simulink model "Citation_FlightGear_v2"  (R2026a)
settings: Solver=ode5  StopTime=40  FixedStep=0.01  EnableMultiTasking=on
InitFcn:
  | run('initcit.m')
  | run('id_init.m')
values from neighbouring files (symbols this model uses):
  cv1 = 20000    [gear_params.m]
  cv2 = cv1    (= 20000)    [gear_params.m]
  cv3 = 4000    [gear_params.m]
  cv4 = 20000    [gear_params.m]
  deltagmax1 = 0.25    [gear_params.m]
  deltagmax2 = deltagmax1    (= 0.25)    [gear_params.m]
  deltagmax3 = 0.24    [gear_params.m]
  deltagmax4 = 0.02    [gear_params.m]
  kt1 = 525020    [gear_params.m]
  kt2 = kt1    (= 525020)    [gear_params.m]
  kt3 = 457050    [gear_params.m]
  murol = 0.03*10    (= 0.3)    [gear_params.m]
  P1 = 2000    [gear_params.m]
  P2 = P1    (= 2000)    [gear_params.m]
  P3 = 2550    [gear_params.m]
  P4 = 40000    [gear_params.m]
  PL0 = 10000*eye(6)    [id_init.m]
  PM0 = 10000*eye(4)    [id_init.m]
  PN0 = 10000*eye(6)    [id_init.m]
  PX0 = 10000*eye(5)    [id_init.m]
  PY0 = 10000*eye(6)    [id_init.m]
  PZ0 = 10000*eye(4)    [id_init.m]
  thetaL0 = zeros(6,1)    [id_init.m]
  thetaM0 = zeros(4,1)    [id_init.m]
  thetaN0 = zeros(6,1)    [id_init.m]
  thetaX0 = zeros(5,1)    [id_init.m]
  thetaY0 = zeros(6,1)    [id_init.m]
  thetaZ0 = zeros(4,1)    [id_init.m]
  TL = 7.0875e-06    [id_init.m]    (also in plot_comparison_step_4.m = T_var(4))
  TM = 3.2564e-06    [id_init.m]    (also in plot_comparison_step_4.m = T_var(5))
  TN = 5.4692e-07    [id_init.m]    (also in plot_comparison_step_4.m = T_var(6))
  TX = 2.2784e-06    [id_init.m]    (also in plot_comparison_step_4.m = T_var(1))
  TY = 8.0633e-07    [id_init.m]    (also in plot_comparison_step_4.m = T_var(2))
  TZ = 2.8004e-05    [id_init.m]    (also in plot_comparison_step_4.m = T_var(3))
  xl1 = xcg-6.858    [gear_params.m]
  xl2 = xcg-6.858    [gear_params.m]
  xl3 = xcg-2.0752    [gear_params.m]
  xl4 = xcg-12.742    [gear_params.m]
  yl1 = 1.918    [gear_params.m]
  yl2 = -1.918    [gear_params.m]
  yl3 = 0    [gear_params.m]
  yl4 = 0    [gear_params.m]
  zl1 = zcg-1.701    [gear_params.m]
  zl2 = zcg-1.701    [gear_params.m]
  zl3 = zcg-1.7488    [gear_params.m]
  zl4 = zcg-2.78    [gear_params.m]
undefined symbols (not defined in the file or in its folder): chord, Deng, ealphag, ealphas, g0, hDME, hGS, lh, massinit, matbuaf, matdaf, matdam, matdbbf, matdeaf, matdgaf, matdqaf, matduaf, matdwaw, matedhr, mateif, matelhr, matemhr, matemv1, matemv2, matemve, matetam, mateuaf, matfaaf, matfaxl, matff, matibaf, matibb, matibmh, matipaf, matipmh, matiraf, matiuaf, matiwaf, matlaf, matlam, matleaf, matleam, matlgaf, matlqaf, matluaf, matmaaf, matmaam, matmaf, matmam, matmbbf, matmeaf, matmeam, matmgaf, matmqaf, matmrbr, matn1d, matn2d, matnbab, matnbaf, matnbmh ... (+53)
libraries: simulink x12, aerolibfltsims x3, aerolibconvert2 x2, aerolibobsolete x1, aerolibanimutils x1
(part 4 of 5)

== system Citation_FlightGear_v2/Cessna Citation 500/Citation model DASMAT/AIRCRAFT MODEL/AFM/Aeromod/SubSystem/model/CLLCAL ==
  in_1 : Inport
  Abs : Abs
  CIBAB : Subsystem  mask(3-D Table Lookup){xindex=matibb(2:5,1), yindex=matibb(1,2:4), zindex=matibb(1,5:7), table=matibb(2:5,2:10)}
      mask prompts: xindex "X Index"; yindex "Y Index"; zindex "Z Index"
      mask help:
      | Three Dimensional Table Lookup
      | The first, second and third input corresponds to the X,Y and Z Index
      mask Help: This block returns a linearly interpolated intersection from the table using the X index (which corresponds to the rows of the table), the Y index (which corresponds to the columns of the table) and the Z index.  Extrapolation is used.
      mask Display: plot(-10,-10,110,110,[90,50,10],[90,40,30],[90,50,10],[50,26,20],[90,50,10],[22,13,10])
  CIBAF : Lookup2D  RowIndex=matibaf(2:4,1)  ColumnIndex=matibaf(1,2:4)  Table=matibaf(2:4,2:4)
  CIBMH : Lookup2D  RowIndex=matibmh(2:10,1)  ColumnIndex=matibmh(1,2:10)  Table=matibmh(2:10,2:10)
  CIPAF : Lookup2D  RowIndex=matipaf(2:3,1)  ColumnIndex=matipaf(1,2:3)  Table=matipaf(2:3,2:3)
  CIPMH : Lookup2D  RowIndex=matipmh(2:10,1)  ColumnIndex=matipmh(1,2:10)  Table=matipmh(2:10,2:10)
  CIRAF : Lookup2D  RowIndex=matiraf(2:4,1)  ColumnIndex=matiraf(1,2:4)  Table=matiraf(2:4,2:4)
  CIRUAF : Lookup2D  RowIndex=matiuaf(2:3,1)  ColumnIndex=matiuaf(1,2:3)  Table=matiuaf(2:3,2:3)
  CIRUMH : Lookup2D  RowIndex=matrumh(2:10,1)  ColumnIndex=matrumh(1,2:10)  Table=matrumh(2:10,2:10)
  CIWAF : Lookup2D  RowIndex=matiwaf(2:3,1)  ColumnIndex=matiwaf(1,2:3)  Table=matiwaf(2:3,2:3)
  CIWTAM : Lookup2D  RowIndex=matwtam(2:3,1)  ColumnIndex=matwtam(1,2:3)  Table=matwtam(2:3,2:3)
  CLL : Sum  Inputs=+++++++  InputSameDT=on  SaturateOnIntegerOverflow=on  OutDataTypeStr=Inherit: Same as first input
  CLLB : Product  InputSameDT=on  SaturateOnIntegerOverflow=on  OutDataTypeStr=Inherit: Same as first input
  CLLDA : Product  InputSameDT=on  SaturateOnIntegerOverflow=on  OutDataTypeStr=Inherit: Same as first input
  CLLDR : Product  InputSameDT=on  SaturateOnIntegerOverflow=on  OutDataTypeStr=Inherit: Same as first input
  CLLGE : Product  Inputs=3  InputSameDT=on  SaturateOnIntegerOverflow=on  OutDataTypeStr=Inherit: Same as first input
  CLLGUST : Mux  Inputs=8
  CLLP : Product  InputSameDT=on  SaturateOnIntegerOverflow=on  OutDataTypeStr=Inherit: Same as first input
  CLLR : Product  InputSameDT=on  SaturateOnIntegerOverflow=on  OutDataTypeStr=Inherit: Same as first input
  CLLTRIM : Product  InputSameDT=on  SaturateOnIntegerOverflow=on  OutDataTypeStr=Inherit: Same as first input
  Demux1 : Demux  Outputs=[1 1 1 1 1 1 1 1 1 1 1 1 1 1 1 1 1 1]
      settings: DisplayOption=none
  LFACT : Subsystem
  LROLL : Lookup  InputValues=mateif(1,:)  Table=mateif(2,:)
  Sum : Sum  Inputs=+++  InputSameDT=on  SaturateOnIntegerOverflow=on  OutDataTypeStr=Inherit: Same as first input
  Sum1 : Sum  InputSameDT=on  SaturateOnIntegerOverflow=on  OutDataTypeStr=Inherit: Same as first input
  Sum2 : Sum  InputSameDT=on  SaturateOnIntegerOverflow=on  OutDataTypeStr=Inherit: Same as first input
  Terminator_{1..7} (7 alike) : Terminator
  "neg " : Gain  Gain=-1  SaturateOnIntegerOverflow=on  OutDataTypeStr=Inherit: Same as input  ParamDataTypeStr=Inherit: Same as input
  zero : Constant  Value=0
  out_1 : Outport
  out_2 : Outport  Port=2
  wires:
  Demux1/18 -> Terminator_7/1
  Demux1/16 -> Terminator_6/1
  Demux1/15 -> Terminator_5/1
  Demux1/13 -> Terminator_4/1
  Demux1/11 -> Terminator_3/1
  Demux1/8 -> Terminator_2/1
  Demux1/2 -> Terminator_1/1
  Sum/1 -> CLLGUST/3, CLLB/2
  LFACT/1(LFACT) -> CLLGE/3
  LROLL/1 -> CLLGE/2
  CLL/1 -> out_1/1
  CLLB/1 -> CLL/1
  CIWTAM/1 -> CLLTRIM/2
  CIWAF/1 -> CLLDA/2
  Sum1/1 -> CLLDR/2
  CIRUMH/1 -> Sum1/2
  Abs/1 -> CIBAB/1(x0)
  CIRUAF/1 -> Sum1/1
  CIBAF/1 -> Sum/1
  CIPAF/1 -> Sum2/1
  CIPMH/1 -> Sum2/2
  Demux1/14 -> CIBAF/1, CIRUAF/1, CIRAF/1, LROLL/1, CIPAF/1, CIWAF/1, CIBAB/3(z0)
  Demux1/5 -> CLLB/1, Abs/1, CLLGE/1
  Demux1/4 -> CIWAF/2, CIRUAF/2, CIPAF/2, CIRAF/2, CIWTAM/2, CIBAB/2(y0), CIBAF/2
  zero/1 -> CLLGUST/2, CLLGUST/5, CLLGUST/6, CLLGUST/4, CLLGUST/1
  CLLGUST/1 -> out_2/1
  CIRAF/1 -> "neg "/1, CLLR/2
  Sum2/1 -> CLLGUST/8, CLLP/2
  "neg "/1 -> CLLGUST/7
  in_1/1 -> Demux1/1
  CLLGE/1 -> CLL/7
  CLLR/1 -> CLL/6
  CLLTRIM/1 -> CLL/4
  CLLDA/1 -> CLL/2
  Demux1/12 -> CLLTRIM/1
  Demux1/10 -> CLLDR/1
  Demux1/9 -> CLLDA/1
  Demux1/1 -> CLLP/1
  Demux1/3 -> CLLR/1
  CIBMH/1 -> Sum/2
  CIBAB/1(out_1) -> Sum/3
  Demux1/17 -> CIRUMH/2, CIWTAM/1, CIPMH/2, CIBMH/2
  Demux1/6 -> CIRUMH/1, CIPMH/1, CIBMH/1
  Demux1/7 -> LFACT/1(hcg)
  CLLP/1 -> CLL/5
  CLLDR/1 -> CLL/3

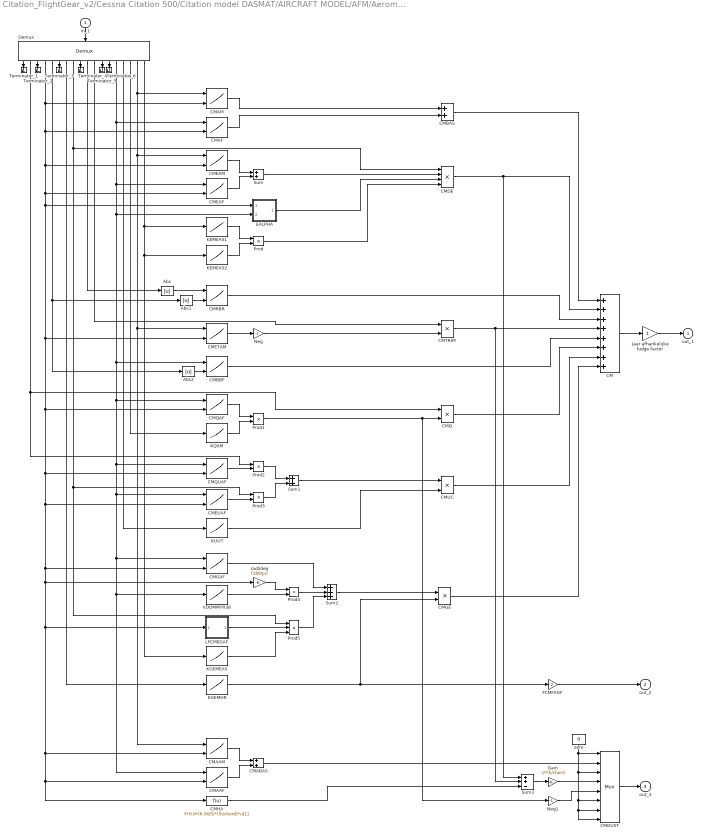
== system Citation_FlightGear_v2/Cessna Citation 500/Citation model DASMAT/AIRCRAFT MODEL/AFM/Aeromod/SubSystem/model/CMCAL ==
  in_1 : Inport
  Abs : Abs
  Abs1 : Abs
  Abs2 : Abs
  CM : Sum  Inputs=++++++++  InputSameDT=on  SaturateOnIntegerOverflow=on  OutDataTypeStr=Inherit: Same as first input
  CMAAF : Lookup2D  RowIndex=matmaaf(2:22,1)  ColumnIndex=matmaaf(1,2:22)  Table=matmaaf(2:22,2:22)
  CMAAM : Lookup2D  RowIndex=matmaam(2:22,1)  ColumnIndex=matmaam(1,2:22)  Table=matmaam(2:22,2:22)
  CMABAS : Sum  InputSameDT=on  SaturateOnIntegerOverflow=on  OutDataTypeStr=Inherit: Same as first input
  CMAF : Lookup2D  RowIndex=matmaf(2:23,1)  ColumnIndex=matmaf(1,2:23)  Table=matmaf(2:23,2:23)
  "CMAM " : Lookup2D  RowIndex=matmam(2:23,1)  ColumnIndex=matmam(1,2:23)  Table=matmam(2:23,2:23)
  CMBAS : Sum  InputSameDT=on  SaturateOnIntegerOverflow=on  OutDataTypeStr=Inherit: Same as first input
  CMBBF : Lookup2D  RowIndex=matmbbf(2:18,1)  ColumnIndex=matmbbf(1,2:18)  Table=matmbbf(2:18,2:18)
  CMDE : Product  Inputs=4  InputSameDT=on  SaturateOnIntegerOverflow=on  OutDataTypeStr=Inherit: Same as first input
  CMEAF : Lookup2D  RowIndex=matmeaf(2:23,1)  ColumnIndex=matmeaf(1,2:23)  Table=matmeaf(2:23,2:23)
  CMEAM : Lookup2D  RowIndex=matmeam(2:23,1)  ColumnIndex=matmeam(1,2:23)  Table=matmeam(2:23,2:23)
  CMETAM : Lookup2D  RowIndex=matetam(2:3,1)  ColumnIndex=matetam(1,2:3)  Table=matetam(2:3,2:3)
  CMEUAF : Lookup2D  RowIndex=mateuaf(2:23,1)  ColumnIndex=mateuaf(1,2:23)  Table=mateuaf(2:23,2:23)
  CMGAF : Lookup2D  RowIndex=matmgaf(2:4,1)  ColumnIndex=matmgaf(1,2:4)  Table=matmgaf(2:4,2:4)
  CMGE : Product  InputSameDT=on  SaturateOnIntegerOverflow=on  OutDataTypeStr=Inherit: Same as first input
  CMGUST : Mux  Inputs=8
  CMHA : Fcn  Expr=5*0.9*(6.56/S)*(lh/chord)*u[1]
  CMQ : Product  InputSameDT=on  SaturateOnIntegerOverflow=on  OutDataTypeStr=Inherit: Same as first input
  CMQAF : Lookup2D  RowIndex=matmqaf(2:23,1)  ColumnIndex=matmqaf(1,2:23)  Table=matmqaf(2:23,2:23)
  CMQUAF : Lookup2D  RowIndex=matquaf(2:23,1)  ColumnIndex=matquaf(1,2:23)  Table=matquaf(2:23,2:23)
  CMRBR : Lookup2D  RowIndex=matmrbr(2:3,1)  ColumnIndex=matmrbr(1,2:3)  Table=matmrbr(2:3,2:3)
  CMTRIM : Product  InputSameDT=on  SaturateOnIntegerOverflow=on  OutDataTypeStr=Inherit: Same as first input
  CMUC : Product  InputSameDT=on  SaturateOnIntegerOverflow=on  OutDataTypeStr=Inherit: Same as first input
  Demux : Demux  Outputs=[1 1 1 1 1 1 1 1 1 1 1 1 1 1 1 1 1 1]
      settings: DisplayOption=none
  EALPHA : Subsystem
  FCMFAGF : Gain  Gain=-2  SaturateOnIntegerOverflow=on  OutDataTypeStr=Inherit: Same as input  ParamDataTypeStr=Inherit: Same as input
  Gain : Gain  Gain=-2*lh/chord  SaturateOnIntegerOverflow=on  OutDataTypeStr=Inherit: Same as input  ParamDataTypeStr=Inherit: Same as input
  Jaar afhankelijke fudge factor : Gain
  KEMEAS1 : Lookup  InputValues=matemv1(1,:)  Table=matemv1(2,:)
  KEMEAS2 : Lookup  InputValues=matemv2(1,:)  Table=matemv2(2,:)
  KGEMEAS : Lookup  InputValues=matemve(1,:)  Table=matemve(2,:)
  KGEMHR : Lookup  InputValues=matemhr(1,:)  Table=matemhr(2,:)
  KQXM : Lookup  InputValues=matqxm(1,:)  Table=matqxm(2,:)
  KUUT : Lookup  InputValues=matuut(1,:)  Table=matuut(2,:)
  LFCMEGAF : Subsystem
  "Neg " : Gain  Gain=-1  SaturateOnIntegerOverflow=on  OutDataTypeStr=Inherit: Same as input  ParamDataTypeStr=Inherit: Same as input
  Neg1 : Gain  Gain=-1  SaturateOnIntegerOverflow=on  OutDataTypeStr=Inherit: Same as input  ParamDataTypeStr=Inherit: Same as input
  Prod{,1..4} (5 alike) : Product  InputSameDT=on  SaturateOnIntegerOverflow=on  OutDataTypeStr=Inherit: Same as first input
  Prod5 : Product  Inputs=3  InputSameDT=on  SaturateOnIntegerOverflow=on  OutDataTypeStr=Inherit: Same as first input
  Sum : Sum  InputSameDT=on  SaturateOnIntegerOverflow=on  OutDataTypeStr=Inherit: Same as first input
  Sum1 : Sum  InputSameDT=on  SaturateOnIntegerOverflow=on  OutDataTypeStr=Inherit: Same as first input
  Sum2 : Sum  Inputs=+++  InputSameDT=on  SaturateOnIntegerOverflow=on  OutDataTypeStr=Inherit: Same as first input
  Sum3 : Sum  Inputs=++-  InputSameDT=on  SaturateOnIntegerOverflow=on  OutDataTypeStr=Inherit: Same as first input
  Terminator_{1..6} (6 alike) : Terminator
  VDOMMYR38 : Lookup  InputValues=vdommyr38(1,:)  Table=vdommyr38(2,:)
  rad2deg : Gain  Gain=(180/pi)  SaturateOnIntegerOverflow=on  OutDataTypeStr=Inherit: Same as input  ParamDataTypeStr=Inherit: Same as input
  zero : Constant  Value=0
  out_1 : Outport
  out_2 : Outport  Port=2
  "out_3 " : Outport  Port=3
  wires:
  Demux/13 -> Terminator_6/1
  Demux/12 -> Terminator_5/1
  Demux/9 -> Terminator_4/1
  Demux/6 -> Terminator_3/1
  Demux/3 -> Terminator_2/1
  Demux/1 -> Terminator_1/1
  Neg1/1 -> CMGUST/5
  CMABAS/1 -> CMGUST/2
  CMHA/1 -> Sum3/3
  CMGAF/1 -> Sum2/1
  Prod4/1 -> Sum2/2
  VDOMMYR38/1 -> Prod4/2
  CMQUAF/1 -> Prod2/2
  EALPHA/1(EALPHA) -> CMDE/3
  CMBAS/1 -> CM/1
  "CMAM "/1 -> CMBAS/1
  Abs/1 -> CMRBR/1
  Abs2/1 -> CMBBF/2
  KUUT/1 -> CMUC/2
  Sum1/1 -> CMUC/1
  Demux/14 -> CMAF/1, CMEAF/1, EALPHA/2(deltaf), CMQAF/1, CMQUAF/1, CMGAF/1, VDOMMYR38/1, CMAAF/1, CMEUAF/1, CMBBF/1
  Sum/1 -> CMDE/2
  Demux/8 -> CMDE/1, Prod3/1, Prod5/1
  Prod/1 -> CMDE/4
  Demux/18 -> KEMEAS1/1, KEMEAS2/1, KGEMEAS/1
  Demux/2 -> CMQ/1, Prod2/1
  CMETAM/1 -> "Neg "/1
  "Neg "/1 -> CMTRIM/2
  CMEUAF/1 -> Prod3/2
  Sum3/1 -> Gain/1
  Prod2/1 -> Sum1/1
  Sum2/1 -> CMGE/1
  Demux/4 -> "CMAM "/2, CMEAM/2, CMEAF/2, EALPHA/1(alpha), CMQAF/2, CMQUAF/2, CMEUAF/2, CMGAF/2, rad2deg/1, CMAAF/2, CMHA/1, CMAAM/2, LFCMEGAF/1(alpha), CMETAM/2, CMAF/2
  Demux/17 -> "CMAM "/1, CMEAM/1, CMETAM/1, CMAAM/1
  CMUC/1 -> CM/7
  CM/1 -> Jaar afhankelijke fudge factor/1
  CMGE/1 -> CM/8
  Prod1/1 -> Neg1/1, CMQ/2
  FCMFAGF/1 -> out_2/1
  CMGUST/1 -> "out_3 "/1
  Gain/1 -> CMGUST/4
  zero/1 -> CMGUST/6, CMGUST/7, CMGUST/8, CMGUST/3, CMGUST/1
  in_1/1 -> Demux/1
  Abs1/1 -> CMRBR/2
  Demux/5 -> Abs1/1, Abs2/1
  CMQAF/1 -> Prod1/1
  Prod3/1 -> Sum1/2
  CMRBR/1 -> CM/3
  CMQ/1 -> CM/6
  CMBBF/1 -> CM/5
  CMTRIM/1 -> Sum3/2, CM/4
  CMDE/1 -> Sum3/1, CM/2
  CMAF/1 -> CMBAS/2
  CMEAM/1 -> Sum/1
  CMEAF/1 -> Sum/2
  KQXM/1 -> Prod1/2
  CMAAM/1 -> CMABAS/1
  CMAAF/1 -> CMABAS/2
  Demux/16 -> KQXM/1
  Demux/15 -> KUUT/1
  Demux/11 -> CMTRIM/1
  Demux/10 -> Abs/1
  Demux/7 -> KGEMHR/1
  KEMEAS1/1 -> Prod/1
  KEMEAS2/1 -> Prod/2
  LFCMEGAF/1(LFCMEGAF) -> Prod5/2
  KGEMEAS/1 -> Prod5/3
  rad2deg/1 -> Prod4/1
  Prod5/1 -> Sum2/3
  KGEMHR/1 -> FCMFAGF/1, CMGE/2
  Jaar afhankelijke fudge factor/1 -> out_1/1

== system Citation_FlightGear_v2/Cessna Citation 500/Citation model DASMAT/AIRCRAFT MODEL/AFM/Aeromod/SubSystem/model/CNCAL ==
  in_1 : Inport
  Abs : Abs
  CN : Sum  Inputs=++++++  InputSameDT=on  SaturateOnIntegerOverflow=on  OutDataTypeStr=Inherit: Same as first input
  CNB : Product  InputSameDT=on  SaturateOnIntegerOverflow=on  OutDataTypeStr=Inherit: Same as first input
  CNBAB : Lookup2D  RowIndex=matnbab(2:5,1)  ColumnIndex=matnbab(1,2:5)  Table=matnbab(2:5,2:5)
  CNBAF : Lookup2D  RowIndex=matnbaf(2:3,1)  ColumnIndex=matnbaf(1,2:3)  Table=matnbaf(2:3,2:3)
  CNBMH : Lookup2D  RowIndex=matnbmh(2:10,1)  ColumnIndex=matnbmh(1,2:10)  Table=matnbmh(2:10,2:10)
  CNDA : Product  InputSameDT=on  SaturateOnIntegerOverflow=on  OutDataTypeStr=Inherit: Same as first input
  CNDR : Product  InputSameDT=on  SaturateOnIntegerOverflow=on  OutDataTypeStr=Inherit: Same as first input
  CNGUST : Mux  Inputs=8
  CNP : Product  InputSameDT=on  SaturateOnIntegerOverflow=on  OutDataTypeStr=Inherit: Same as first input
  CNPAF : Lookup2D  RowIndex=matnpaf(2:4,1)  ColumnIndex=matnpaf(1,2:4)  Table=matnpaf(2:4,2:4)
  CNPMH : Lookup2D  RowIndex=matnpmh(2:10,1)  ColumnIndex=matnpmh(1,2:10)  Table=matnpmh(2:10,2:10)
  CNR : Product  InputSameDT=on  SaturateOnIntegerOverflow=on  OutDataTypeStr=Inherit: Same as first input
  CNRAF : Lookup2D  RowIndex=matnraf(2:3,1)  ColumnIndex=matnraf(1,2:3)  Table=matnraf(2:3,2:3)
  CNRTAM : Lookup2D  RowIndex=matrtam(2:3,1)  ColumnIndex=matrtam(1,2:3)  Table=matrtam(2:3,2:3)
  CNRUAF : Lookup2D  RowIndex=matnuaf(2:3,1)  ColumnIndex=matnuaf(1,2:3)  Table=matnuaf(2:3,2:3)
  CNTRIM : Product  InputSameDT=on  SaturateOnIntegerOverflow=on  OutDataTypeStr=Inherit: Same as first input
  CNWAF : Lookup2D  RowIndex=matnwaf(2:4,1)  ColumnIndex=matnwaf(1,2:4)  Table=matnwaf(2:4,2:4)
  CNWMH : Lookup2D  RowIndex=matnwmh(2:10,1)  ColumnIndex=matnwmh(1,2:10)  Table=matnwmh(2:10,2:10)
  Demux : Demux  Outputs=[1 1 1 1 1 1 1 1 1 1 1 1 1 1 1 1 1 1]
      settings: DisplayOption=none
  Neg : Gain  Gain=-1  SaturateOnIntegerOverflow=on  OutDataTypeStr=Inherit: Same as input  ParamDataTypeStr=Inherit: Same as input
  Sum : Sum  Inputs=+++  InputSameDT=on  SaturateOnIntegerOverflow=on  OutDataTypeStr=Inherit: Same as first input
  Sum1 : Sum  InputSameDT=on  SaturateOnIntegerOverflow=on  OutDataTypeStr=Inherit: Same as first input
  Sum2 : Sum  InputSameDT=on  SaturateOnIntegerOverflow=on  OutDataTypeStr=Inherit: Same as first input
  Terminator_{1..8} (8 alike) : Terminator
  zero : Constant  Value=0
  out_1 : Outport
  "out_2 " : Outport  Port=2
  wires:
  Demux/18 -> Terminator_8/1
  Demux/16 -> Terminator_7/1
  Demux/15 -> Terminator_6/1
  Demux/12 -> Terminator_5/1
  Demux/11 -> Terminator_4/1
  Demux/8 -> Terminator_3/1
  Demux/7 -> Terminator_2/1
  Demux/2 -> Terminator_1/1
  Sum/1 -> CNGUST/3, CNB/2
  CNR/1 -> CN/6
  CNB/1 -> CN/1
  CNDR/1 -> CN/3
  CNRTAM/1 -> CNTRIM/2
  CNRUAF/1 -> CNDR/2
  Sum1/1 -> CNDA/2
  Abs/1 -> CNBAB/1
  CN/1 -> out_1/1
  Demux/4 -> CNBAF/2, CNBAB/2, CNWAF/2, CNRTAM/2, CNPAF/2, CNRAF/2, CNRUAF/2
  Demux/5 -> CNB/1, Abs/1
  CNWAF/1 -> Sum1/1
  CNWMH/1 -> Sum1/2
  Demux/14 -> CNBAF/1, CNWAF/1, CNPAF/1, CNRAF/1, CNRUAF/1
  Demux/6 -> CNBMH/1, CNWMH/1, CNPMH/1
  CNBAF/1 -> Sum/1
  CNPAF/1 -> Sum2/1
  CNPMH/1 -> Sum2/2
  CNRAF/1 -> Neg/1, CNR/2
  Neg/1 -> CNGUST/7
  CNGUST/1 -> "out_2 "/1
  zero/1 -> CNGUST/2, CNGUST/4, CNGUST/5, CNGUST/6, CNGUST/1
  in_1/1 -> Demux/1
  Demux/17 -> CNBMH/2, CNRTAM/1, CNPMH/2, CNWMH/2
  CNDA/1 -> CN/2
  CNP/1 -> CN/5
  CNTRIM/1 -> CN/4
  Sum2/1 -> CNGUST/8, CNP/2
  Demux/13 -> CNTRIM/1
  Demux/10 -> CNDR/1
  Demux/9 -> CNDA/1
  Demux/1 -> CNP/1
  Demux/3 -> CNR/1
  CNBMH/1 -> Sum/2
  CNBAB/1 -> Sum/3

== system Citation_FlightGear_v2/Cessna Citation 500/Citation model DASMAT/AIRCRAFT MODEL/AFM/Aeromod/SubSystem/model/CXGUST CZGUST ==
  CD : Inport
  CL : Inport  Port=2
  x : Inport  Port=3
  gust : Inport  Port=4
  CDalpha : Constant  Value=0.57
  CLalpha : Constant  Value=5.51
  CX/ ag : Sum  Inputs=+-  InputSameDT=on  SaturateOnIntegerOverflow=on  OutDataTypeStr=Inherit: Same as first input
  CX/ ug : Gain  Gain=2  SaturateOnIntegerOverflow=on  OutDataTypeStr=Inherit: Same as input  ParamDataTypeStr=Inherit: Same as input
  CXGUST : DotProduct  OutDataTypeStr=Inherit: Inherit via internal rule
  CXbody : Fcn  Expr=-u[13]*cos(u[5])+u[14]*sin(u[5])
  CZ/ ag : Gain  Gain=-1  SaturateOnIntegerOverflow=on  OutDataTypeStr=Inherit: Same as input  ParamDataTypeStr=Inherit: Same as input
  CZ/ ug : Gain  Gain=2  SaturateOnIntegerOverflow=on  OutDataTypeStr=Inherit: Same as input  ParamDataTypeStr=Inherit: Same as input
  CZGUST : DotProduct  OutDataTypeStr=Inherit: Inherit via internal rule
  CZbody : Fcn  Expr=-u[14]*cos(u[5])-u[13]*sin(u[5])
  Mux : Mux  Inputs=[12 1 1]
  Mux1 : Mux  Inputs=8
  Mux2 : Mux  Inputs=8
  zero : Constant  Value=0
  zero1 : Constant  Value=0
  "out_1 " : Outport
  "out_2 " : Outport  Port=2
  wires:
  zero1/1 -> Mux2/3, Mux2/7, Mux2/8, Mux2/6, Mux2/5, Mux2/4
  CZ/ ag/1 -> Mux2/2
  zero/1 -> Mux1/3, Mux1/7, Mux1/8, Mux1/6, Mux1/5, Mux1/4
  CX/ ag/1 -> Mux1/2
  CZGUST/1 -> "out_2 "/1
  CXGUST/1 -> "out_1 "/1
  gust/1 -> CZGUST/2, CXGUST/2
  Mux2/1 -> CZGUST/1
  Mux1/1 -> CXGUST/1
  Mux/1 -> CXbody/1, CZbody/1
  CL/1 -> CX/ ag/1, Mux/3
  CD/1 -> Mux/2
  x/1 -> Mux/1
  CDalpha/1 -> CX/ ag/2
  CLalpha/1 -> CZ/ ag/1
  CZbody/1 -> CZ/ ug/1
  CX/ ug/1 -> Mux1/1
  CXbody/1 -> CX/ ug/1
  CZ/ ug/1 -> Mux2/1

== system Citation_FlightGear_v2/Cessna Citation 500/Citation model DASMAT/AIRCRAFT MODEL/AFM/Aeromod/SubSystem/model/CYCAL ==
  in_1 : Inport
  Abs : Abs
  CY : Sum  Inputs=+++++  InputSameDT=on  SaturateOnIntegerOverflow=on  OutDataTypeStr=Inherit: Same as first input
  CY/ BETA : Sum  InputSameDT=on  SaturateOnIntegerOverflow=on  OutDataTypeStr=Inherit: Same as first input
  CYBAB : Lookup2D  RowIndex=matybab(2:5,1)  ColumnIndex=matybab(1,2:5)  Table=matybab(2:5,2:5)
  CYBAF : Lookup2D  RowIndex=matybaf(2:3,1)  ColumnIndex=matybaf(1,2:3)  Table=matybaf(2:3,2:3)
  CYBETA : Product  InputSameDT=on  SaturateOnIntegerOverflow=on  OutDataTypeStr=Inherit: Same as first input
  CYBUAF : Lookup2D  RowIndex=matbuaf(2:3,1)  ColumnIndex=matbuaf(1,2:3)  Table=matbuaf(2:3,2:3)
  CYBUC : Product  InputSameDT=on  SaturateOnIntegerOverflow=on  OutDataTypeStr=Inherit: Same as first input
  CYDA : Product  InputSameDT=on  SaturateOnIntegerOverflow=on  OutDataTypeStr=Inherit: Same as first input
  CYDR : Product  Inputs=3  InputSameDT=on  SaturateOnIntegerOverflow=on  OutDataTypeStr=Inherit: Same as first input
  CYGUST : Mux  Inputs=8
  CYR : Product  InputSameDT=on  SaturateOnIntegerOverflow=on  OutDataTypeStr=Inherit: Same as first input
  CYRAF : Lookup2D  RowIndex=matyraf(2:3,1)  ColumnIndex=matyraf(1,2:3)  Table=matyraf(2:3,2:3)
  CYRUAF : Lookup2D  RowIndex=matyuaf(2:3,1)  ColumnIndex=matyuaf(1,2:3)  Table=matyuaf(2:3,2:3)
  CYWAF : Lookup2D  RowIndex=matywaf(2:3,1)  ColumnIndex=matywaf(1,2:3)  Table=matywaf(2:3,2:3)
  Demux : Demux  Outputs=[1 1 1 1 1 1 1 1 1 1 1 1 1 1 1 1 1 1]
      settings: DisplayOption=none
  KUUT : Lookup  InputValues=matuut(1,:)  Table=matuut(2,:)
  LSFACT : Subsystem
  Prod : Product  InputSameDT=on  SaturateOnIntegerOverflow=on  OutDataTypeStr=Inherit: Same as first input
  Sum : Sum  InputSameDT=on  SaturateOnIntegerOverflow=on  OutDataTypeStr=Inherit: Same as first input
  Terminator_{1..11} (11 alike) : Terminator
  zero : Constant  Value=0
  out_1 : Outport
  out_2 : Outport  Port=2
  wires:
  Demux/18 -> Terminator_11/1
  Demux/17 -> Terminator_10/1
  Demux/16 -> Terminator_9/1
  Demux/13 -> Terminator_8/1
  Demux/12 -> Terminator_7/1
  Demux/11 -> Terminator_6/1
  Demux/8 -> Terminator_5/1
  Demux/7 -> Terminator_4/1
  Demux/6 -> Terminator_3/1
  Demux/2 -> Terminator_2/1
  Demux/1 -> Terminator_1/1
  CY/ BETA/1 -> CYGUST/3
  CYBUAF/1 -> Prod/1
  CYBUC/1 -> CY/5
  CYR/1 -> CY/4
  CYBETA/1 -> CY/1
  CYRAF/1 -> CYR/2
  CYWAF/1 -> CYDA/2
  CYBAB/1 -> Sum/2
  CYBAF/1 -> Sum/1
  Abs/1 -> CYBAB/1
  CY/1 -> out_1/1
  KUUT/1 -> Prod/2
  Demux/14 -> CYBAF/1, CYRUAF/1, CYRAF/1, CYBUAF/1, CYWAF/1
  Demux/5 -> CYBETA/1, Abs/1, CYBUC/1
  Demux/4 -> CYBAF/2, CYWAF/2, CYRAF/2, CYBUAF/2, CYRUAF/2, CYBAB/2
  CYGUST/1 -> out_2/1
  zero/1 -> CYGUST/2, CYGUST/7, CYGUST/8, CYGUST/6, CYGUST/5, CYGUST/4, CYGUST/1
  in_1/1 -> Demux/1
  CYRUAF/1 -> CYDR/2
  Demux/10 -> CYDR/1, LSFACT/1(deltar)
  Sum/1 -> CY/ BETA/1, CYBETA/2
  Prod/1 -> CY/ BETA/2, CYBUC/2
  CYDA/1 -> CY/2
  CYDR/1 -> CY/3
  Demux/3 -> CYR/1
  Demux/15 -> KUUT/1
  Demux/9 -> CYDA/1
  LSFACT/1(LSFACT) -> CYDR/3

== system Citation_FlightGear_v2/Cessna Citation 500/Citation model DASMAT/AIRCRAFT MODEL/EFM/Engmod/Citation eng_mod/Subsystem1/JT15 Dynamic ==
  In1 : Inport
  Demux : Demux  Outputs=32
      settings: DisplayOption=none
  Mux : Mux  Inputs=11
  Subsystem : Subsystem
  Out1 : Outport
  wires:
  Demux/32 -> Subsystem/32(Deng)
  Demux/31 -> Subsystem/31(VIAS)
  Demux/30 -> Subsystem/30(VCAS)
  Demux/29 -> Subsystem/29(VEAS)
  Demux/28 -> Subsystem/28(temptot)
  Demux/27 -> Subsystem/27(ptot)
  Demux/26 -> Subsystem/26(qrel)
  Demux/25 -> Subsystem/25(qc)
  Demux/24 -> Subsystem/24(Reynl)
  Demux/23 -> Subsystem/23(qdyn)
  Demux/22 -> Subsystem/22(Mach)
  Demux/21 -> Subsystem/21(Vsound)
  Demux/20 -> Subsystem/20(Hgeopot)
  Demux/19 -> Subsystem/19(hradio)
  Demux/18 -> Subsystem/18(hpress)
  Demux/17 -> Subsystem/17(grav)
  Demux/16 -> Subsystem/16(temp)
  Demux/15 -> Subsystem/15(rho)
  Demux/14 -> Subsystem/14(pstat)
  Demux/13 -> Subsystem/13(ut)
  Demux/12 -> Subsystem/12(ye)
  Demux/11 -> Subsystem/11(xe)
  Demux/10 -> Subsystem/10(he)
  Demux/9 -> Subsystem/9(psi)
  Demux/8 -> Subsystem/8(theta)
  Demux/7 -> Subsystem/7(phi)
  Demux/6 -> Subsystem/6(beta)
  Demux/5 -> Subsystem/5(alpha)
  Demux/4 -> Subsystem/4(VTAS)
  Demux/3 -> Subsystem/3(rbody)
  Demux/2 -> Subsystem/2(qbody)
  Demux/1 -> Subsystem/1(pbody)
  Subsystem/2(FF) -> Mux/2
  Subsystem/3(N1) -> Mux/3
  Subsystem/4(N2) -> Mux/4
  Subsystem/5(N1c) -> Mux/5
  Subsystem/6(N2c) -> Mux/6
  Subsystem/7(WT) -> Mux/7
  Subsystem/8(ITT) -> Mux/8
  Subsystem/9(EGT) -> Mux/9
  Subsystem/10(OILT) -> Mux/10
  Subsystem/11(OILP) -> Mux/11
  Subsystem/1(Tn) -> Mux/1
  In1/1 -> Demux/1
  Mux/1 -> Out1/1

== system Citation_FlightGear_v2/Cessna Citation 500/Citation model DASMAT/AIRCRAFT MODEL/EFM/Engmod/Citation eng_mod/Subsystem1/JT15 Dynamic1 ==
  In1 : Inport
  Demux : Demux  Outputs=32
      settings: DisplayOption=none
  Mux : Mux  Inputs=11
  Subsystem : Subsystem
  Out1 : Outport
  wires:
  Demux/32 -> Subsystem/32(Deng)
  Demux/31 -> Subsystem/31(VIAS)
  Demux/30 -> Subsystem/30(VCAS)
  Demux/29 -> Subsystem/29(VEAS)
  Demux/28 -> Subsystem/28(temptot)
  Demux/27 -> Subsystem/27(ptot)
  Demux/26 -> Subsystem/26(qrel)
  Demux/25 -> Subsystem/25(qc)
  Demux/24 -> Subsystem/24(Reynl)
  Demux/23 -> Subsystem/23(qdyn)
  Demux/22 -> Subsystem/22(Mach)
  Demux/21 -> Subsystem/21(Vsound)
  Demux/20 -> Subsystem/20(Hgeopot)
  Demux/19 -> Subsystem/19(hradio)
  Demux/18 -> Subsystem/18(hpress)
  Demux/17 -> Subsystem/17(grav)
  Demux/16 -> Subsystem/16(temp)
  Demux/15 -> Subsystem/15(rho)
  Demux/14 -> Subsystem/14(pstat)
  Demux/13 -> Subsystem/13(ut)
  Demux/12 -> Subsystem/12(ye)
  Demux/11 -> Subsystem/11(xe)
  Demux/10 -> Subsystem/10(he)
  Demux/9 -> Subsystem/9(psi)
  Demux/8 -> Subsystem/8(theta)
  Demux/7 -> Subsystem/7(phi)
  Demux/6 -> Subsystem/6(beta)
  Demux/5 -> Subsystem/5(alpha)
  Demux/4 -> Subsystem/4(VTAS)
  Demux/3 -> Subsystem/3(rbody)
  Demux/2 -> Subsystem/2(qbody)
  Demux/1 -> Subsystem/1(pbody)
  Subsystem/2(FF) -> Mux/2
  Subsystem/3(N1) -> Mux/3
  Subsystem/4(N2) -> Mux/4
  Subsystem/5(N1c) -> Mux/5
  Subsystem/6(N2c) -> Mux/6
  Subsystem/7(WT) -> Mux/7
  Subsystem/8(ITT) -> Mux/8
  Subsystem/9(EGT) -> Mux/9
  Subsystem/10(OILT) -> Mux/10
  Subsystem/11(OILP) -> Mux/11
  Subsystem/1(Tn) -> Mux/1
  In1/1 -> Demux/1
  Mux/1 -> Out1/1

== system Citation_FlightGear_v2/Cessna Citation 500/Citation model DASMAT/AIRCRAFT MODEL/AFM/Aeromod/SubSystem/model/CDCAL/KBASD ==
  hcg : Inport
  deltaf : Inport  Port=2
  VEAS : Inport  Port=3
  Constant : Constant
  Fcn : Fcn  Expr=0.2-u[1]
  Fcn1 : Fcn  Expr=u[2]*(u[1]*180/pi-15)*0.04*(100-u[3])/30
  Fcn2 : Fcn  Expr=1-0.6*u[1]
  KGEDHR : Lookup  InputValues=matedhr(1,:)  Table=matedhr(2,:)
  Mux : Mux  Inputs=3
  Sat : Saturate  UpperLimit=1  LowerLimit=0
  Switch : Switch
  KBASD : Outport
  wires:
  KGEDHR/1 -> Mux/2
  deltaf/1 -> Mux/1, Fcn/1
  Fcn/1 -> Switch/2
  Constant/1 -> Switch/1
  Switch/1 -> KBASD/1
  VEAS/1 -> Mux/3
  hcg/1 -> KGEDHR/1
  Mux/1 -> Fcn1/1
  Sat/1 -> Fcn2/1
  Fcn1/1 -> Sat/1
  Fcn2/1 -> Switch/3

== system Citation_FlightGear_v2/Cessna Citation 500/Citation model DASMAT/AIRCRAFT MODEL/AFM/Aeromod/SubSystem/model/CLCAL/CLGEAF ==
  alpha : Inport
  deltaf : Inport  Port=2
  Prod : Product  InputSameDT=on  SaturateOnIntegerOverflow=on  OutDataTypeStr=Inherit: Same as first input
  Sat : Saturate  UpperLimit=0.04  LowerLimit=-inf
  Sum : Sum  InputSameDT=on  SaturateOnIntegerOverflow=on  OutDataTypeStr=Inherit: Same as first input
  VDOMMYR37 : Lookup  InputValues=vdommyr37(1,:)  Table=vdommyr37(2,:)
  VDOMMYR40 : Gain  Gain=1.6  SaturateOnIntegerOverflow=on  OutDataTypeStr=Inherit: Same as input  ParamDataTypeStr=Inherit: Same as input
  rad2deg : Gain  Gain=(180/pi)  SaturateOnIntegerOverflow=on  OutDataTypeStr=Inherit: Same as input  ParamDataTypeStr=Inherit: Same as input
  CLGEAF : Outport
  wires:
  VDOMMYR37/1 -> VDOMMYR40/1, Prod/2
  rad2deg/1 -> Prod/1
  Sat/1 -> rad2deg/1
  alpha/1 -> Sat/1
  deltaf/1 -> VDOMMYR37/1
  VDOMMYR40/1 -> Sum/2
  Prod/1 -> Sum/1
  Sum/1 -> CLGEAF/1

== system Citation_FlightGear_v2/Cessna Citation 500/Citation model DASMAT/AIRCRAFT MODEL/AFM/Aeromod/SubSystem/model/CLCAL/SP0 ==
  deltae : Inport
  Abs : Abs
  Fcn : Fcn  Expr=(0.087+0.25*(u[1]-0.087))/(u[1]+1e-11)
  Prod : Product  InputSameDT=on  SaturateOnIntegerOverflow=on  OutDataTypeStr=Inherit: Same as first input
  Sat : Saturate  UpperLimit=1  LowerLimit=-inf
  SP0 : Outport
  wires:
  deltae/1 -> Prod/1, Abs/1
  Sat/1 -> Prod/2
  Fcn/1 -> Sat/1
  Abs/1 -> Fcn/1
  Prod/1 -> SP0/1

== system Citation_FlightGear_v2/Cessna Citation 500/Citation model DASMAT/AIRCRAFT MODEL/AFM/Aeromod/SubSystem/model/CLLCAL/CIBAB ==
  note: 02-11-2000
      | Modified by A. R. Veldhuijzen
      | sftable3.m was replaced with table3.dll
      | X and Y are exchanged in this Mathworks implementation
  x0 : Inport
  y0 : Inport  Port=2
  z0 : Inport  Port=3
  Mux : Mux  Inputs=3
  S-function : S-Function  FunctionName=table3  Parameters=yindex, xindex ,zindex, table  SFunctionDeploymentMode=off  EnableBusSupport=off
  out_1 : Outport
  wires:
  z0/1 -> Mux/3
  y0/1 -> Mux/1
  x0/1 -> Mux/2
  Mux/1 -> S-function/1
  S-function/1 -> out_1/1

== system Citation_FlightGear_v2/Cessna Citation 500/Citation model DASMAT/AIRCRAFT MODEL/AFM/Aeromod/SubSystem/model/CLLCAL/LFACT ==
  hcg : Inport
  Sat : Saturate  UpperLimit=1  LowerLimit=0
  hrunway : Fcn  Expr=1-(u[1]-1)/30
  LFACT : Outport
  wires:
  Sat/1 -> LFACT/1
  hcg/1 -> hrunway/1
  hrunway/1 -> Sat/1

== system Citation_FlightGear_v2/Cessna Citation 500/Citation model DASMAT/AIRCRAFT MODEL/AFM/Aeromod/SubSystem/model/CMCAL/EALPHA ==
  alpha : Inport
  deltaf : Inport  Port=2
  Fcn : Fcn  Expr=1-u[1]*u[2]
  Mux : Mux  Inputs=2
  Sat : Saturate  UpperLimit=1  LowerLimit=0
  Sum : Sum  Inputs=+-  InputSameDT=on  SaturateOnIntegerOverflow=on  OutDataTypeStr=Inherit: Same as first input
  ealphag : Lookup  InputValues=ealphag(1,:)  Table=ealphag(2,:)
  ealphas : Lookup  InputValues=ealphas(1,:)  Table=ealphas(2,:)
  EALPHA : Outport
  wires:
  deltaf/1 -> ealphag/1, ealphas/1
  alpha/1 -> Sum/1
  Mux/1 -> Fcn/1
  ealphag/1 -> Mux/2
  ealphas/1 -> Sum/2
  Sum/1 -> Mux/1
  Fcn/1 -> Sat/1
  Sat/1 -> EALPHA/1

== system Citation_FlightGear_v2/Cessna Citation 500/Citation model DASMAT/AIRCRAFT MODEL/AFM/Aeromod/SubSystem/model/CMCAL/LFCMEGAF ==
  alpha : Inport
  Abs : Abs
  Fcn : Fcn  Expr=1-5*u[1]
  Neg : Gain  Gain=-1  SaturateOnIntegerOverflow=on  OutDataTypeStr=Inherit: Same as input  ParamDataTypeStr=Inherit: Same as input
  Sat : Saturate  UpperLimit=inf  LowerLimit=0.25
  LFCMEGAF : Outport
  wires:
  Fcn/1 -> Sat/1
  alpha/1 -> Abs/1
  Abs/1 -> Fcn/1
  Sat/1 -> Neg/1
  Neg/1 -> LFCMEGAF/1

== system Citation_FlightGear_v2/Cessna Citation 500/Citation model DASMAT/AIRCRAFT MODEL/AFM/Aeromod/SubSystem/model/CYCAL/LSFACT ==
  deltar : Inport
  Abs : Abs
  Fcn : Fcn  Expr=0.06981/u[1]+2*(u[1]-0.06981)
  Sat : Saturate  UpperLimit=inf  LowerLimit=0.06981
  LSFACT : Outport
  wires:
  deltar/1 -> Abs/1
  Abs/1 -> Sat/1
  Sat/1 -> Fcn/1
  Fcn/1 -> LSFACT/1

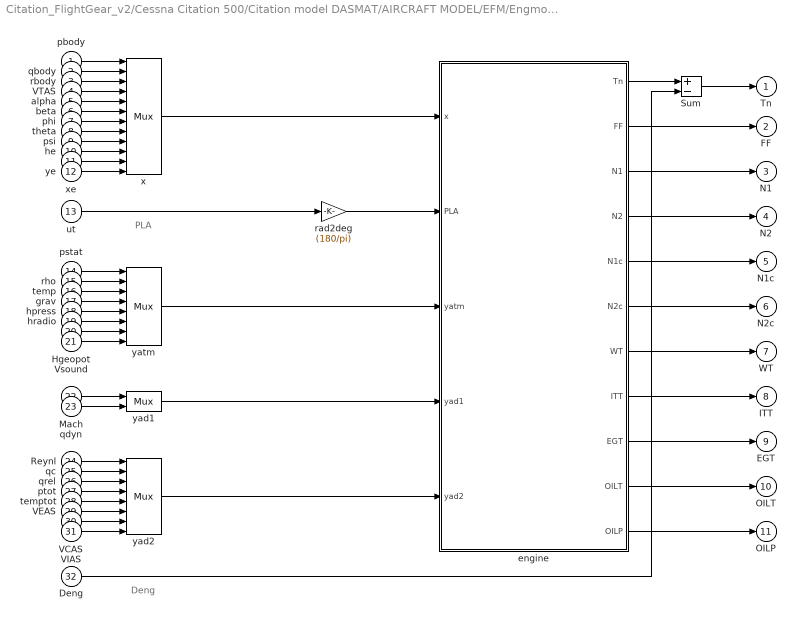
== system Citation_FlightGear_v2/Cessna Citation 500/Citation model DASMAT/AIRCRAFT MODEL/EFM/Engmod/Citation eng_mod/Subsystem1/JT15 Dynamic/Subsystem ==
  note: Deng
  note: PLA
  pbody : Inport
  qbody : Inport  Port=2
  rbody : Inport  Port=3
  VTAS : Inport  Port=4
  alpha : Inport  Port=5
  beta : Inport  Port=6
  phi : Inport  Port=7
  theta : Inport  Port=8
  psi : Inport  Port=9
  he : Inport  Port=10
  xe : Inport  Port=11
  ye : Inport  Port=12
  ut : Inport  Port=13
  pstat : Inport  Port=14
  rho : Inport  Port=15
  temp : Inport  Port=16
  grav : Inport  Port=17
  hpress : Inport  Port=18
  hradio : Inport  Port=19
  Hgeopot : Inport  Port=20
  Vsound : Inport  Port=21
  Mach : Inport  Port=22
  qdyn : Inport  Port=23
  Reynl : Inport  Port=24
  qc : Inport  Port=25
  qrel : Inport  Port=26
  ptot : Inport  Port=27
  temptot : Inport  Port=28
  VEAS : Inport  Port=29
  VCAS : Inport  Port=30
  VIAS : Inport  Port=31
  Deng : Inport  Port=32
  Sum : Sum  Inputs=+-  InputSameDT=on  SaturateOnIntegerOverflow=on  OutDataTypeStr=Inherit: Same as first input
  engine : Subsystem
  rad2deg : Gain  Gain=(180/pi)  SaturateOnIntegerOverflow=on  OutDataTypeStr=Inherit: Same as input  ParamDataTypeStr=Inherit: Same as input
  x : Mux  Inputs=12
  yad1 : Mux  Inputs=2
  yad2 : Mux  Inputs=8
  yatm : Mux  Inputs=8
  Tn : Outport
  FF : Outport  Port=2
  N1 : Outport  Port=3
  N2 : Outport  Port=4
  N1c : Outport  Port=5
  N2c : Outport  Port=6
  WT : Outport  Port=7
  ITT : Outport  Port=8
  EGT : Outport  Port=9
  OILT : Outport  Port=10
  OILP : Outport  Port=11
  wires:
  Deng/1 -> Sum/2
  engine/1(Tn) -> Sum/1
  Sum/1 -> Tn/1
  Vsound/1 -> yatm/8
  engine/11(OILP) -> OILP/1
  engine/10(OILT) -> OILT/1
  rad2deg/1 -> engine/2(PLA)
  ut/1 -> rad2deg/1
  engine/9(EGT) -> EGT/1
  engine/8(ITT) -> ITT/1
  engine/7(WT) -> WT/1
  engine/6(N2c) -> N2c/1
  engine/5(N1c) -> N1c/1
  engine/4(N2) -> N2/1
  engine/3(N1) -> N1/1
  engine/2(FF) -> FF/1
  yad1/1 -> engine/4(yad1)
  yatm/1 -> engine/3(yatm)
  yad2/1 -> engine/5(yad2)
  qdyn/1 -> yad1/2
  Mach/1 -> yad1/1
  Reynl/1 -> yad2/1
  qc/1 -> yad2/2
  VCAS/1 -> yad2/7
  temptot/1 -> yad2/5
  qrel/1 -> yad2/3
  VIAS/1 -> yad2/8
  VEAS/1 -> yad2/6
  ptot/1 -> yad2/4
  ye/1 -> x/12
  xe/1 -> x/11
  he/1 -> x/10
  psi/1 -> x/9
  VTAS/1 -> x/4
  beta/1 -> x/6
  theta/1 -> x/8
  rbody/1 -> x/3
  alpha/1 -> x/5
  phi/1 -> x/7
  qbody/1 -> x/2
  pbody/1 -> x/1
  pstat/1 -> yatm/1
  rho/1 -> yatm/2
  Hgeopot/1 -> yatm/7
  hpress/1 -> yatm/5
  temp/1 -> yatm/3
  hradio/1 -> yatm/6
  grav/1 -> yatm/4
  x/1 -> engine/1(x)

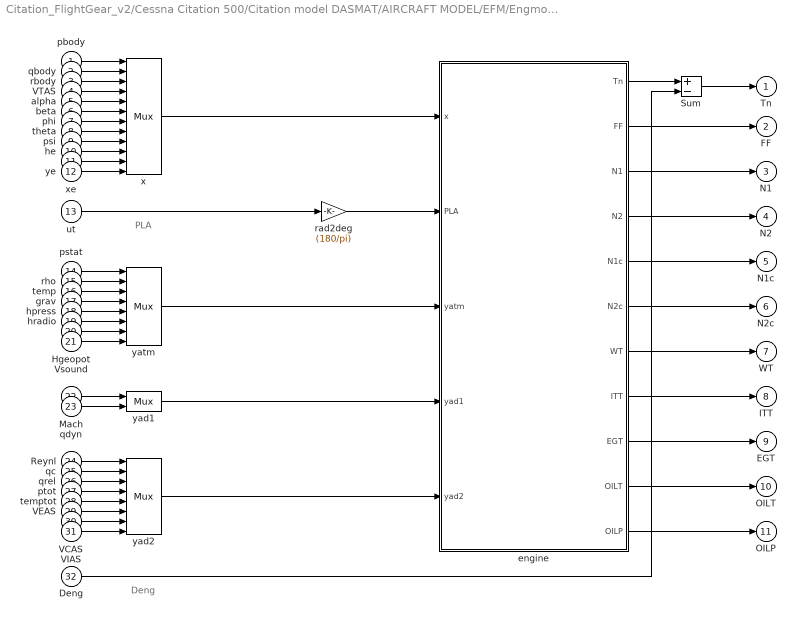
== system Citation_FlightGear_v2/Cessna Citation 500/Citation model DASMAT/AIRCRAFT MODEL/EFM/Engmod/Citation eng_mod/Subsystem1/JT15 Dynamic1/Subsystem ==
  note: Deng
  note: PLA
  pbody : Inport
  qbody : Inport  Port=2
  rbody : Inport  Port=3
  VTAS : Inport  Port=4
  alpha : Inport  Port=5
  beta : Inport  Port=6
  phi : Inport  Port=7
  theta : Inport  Port=8
  psi : Inport  Port=9
  he : Inport  Port=10
  xe : Inport  Port=11
  ye : Inport  Port=12
  ut : Inport  Port=13
  pstat : Inport  Port=14
  rho : Inport  Port=15
  temp : Inport  Port=16
  grav : Inport  Port=17
  hpress : Inport  Port=18
  hradio : Inport  Port=19
  Hgeopot : Inport  Port=20
  Vsound : Inport  Port=21
  Mach : Inport  Port=22
  qdyn : Inport  Port=23
  Reynl : Inport  Port=24
  qc : Inport  Port=25
  qrel : Inport  Port=26
  ptot : Inport  Port=27
  temptot : Inport  Port=28
  VEAS : Inport  Port=29
  VCAS : Inport  Port=30
  VIAS : Inport  Port=31
  Deng : Inport  Port=32
  Sum : Sum  Inputs=+-  InputSameDT=on  SaturateOnIntegerOverflow=on  OutDataTypeStr=Inherit: Same as first input
  engine : Subsystem
  rad2deg : Gain  Gain=(180/pi)  SaturateOnIntegerOverflow=on  OutDataTypeStr=Inherit: Same as input  ParamDataTypeStr=Inherit: Same as input
  x : Mux  Inputs=12
  yad1 : Mux  Inputs=2
  yad2 : Mux  Inputs=8
  yatm : Mux  Inputs=8
  Tn : Outport
  FF : Outport  Port=2
  N1 : Outport  Port=3
  N2 : Outport  Port=4
  N1c : Outport  Port=5
  N2c : Outport  Port=6
  WT : Outport  Port=7
  ITT : Outport  Port=8
  EGT : Outport  Port=9
  OILT : Outport  Port=10
  OILP : Outport  Port=11
  wires:
  Deng/1 -> Sum/2
  engine/1(Tn) -> Sum/1
  Sum/1 -> Tn/1
  Vsound/1 -> yatm/8
  engine/11(OILP) -> OILP/1
  engine/10(OILT) -> OILT/1
  rad2deg/1 -> engine/2(PLA)
  ut/1 -> rad2deg/1
  engine/9(EGT) -> EGT/1
  engine/8(ITT) -> ITT/1
  engine/7(WT) -> WT/1
  engine/6(N2c) -> N2c/1
  engine/5(N1c) -> N1c/1
  engine/4(N2) -> N2/1
  engine/3(N1) -> N1/1
  engine/2(FF) -> FF/1
  yad1/1 -> engine/4(yad1)
  yatm/1 -> engine/3(yatm)
  yad2/1 -> engine/5(yad2)
  qdyn/1 -> yad1/2
  Mach/1 -> yad1/1
  Reynl/1 -> yad2/1
  qc/1 -> yad2/2
  VCAS/1 -> yad2/7
  temptot/1 -> yad2/5
  qrel/1 -> yad2/3
  VIAS/1 -> yad2/8
  VEAS/1 -> yad2/6
  ptot/1 -> yad2/4
  ye/1 -> x/12
  xe/1 -> x/11
  he/1 -> x/10
  psi/1 -> x/9
  VTAS/1 -> x/4
  beta/1 -> x/6
  theta/1 -> x/8
  rbody/1 -> x/3
  alpha/1 -> x/5
  phi/1 -> x/7
  qbody/1 -> x/2
  pbody/1 -> x/1
  pstat/1 -> yatm/1
  rho/1 -> yatm/2
  Hgeopot/1 -> yatm/7
  hpress/1 -> yatm/5
  temp/1 -> yatm/3
  hradio/1 -> yatm/6
  grav/1 -> yatm/4
  x/1 -> engine/1(x)

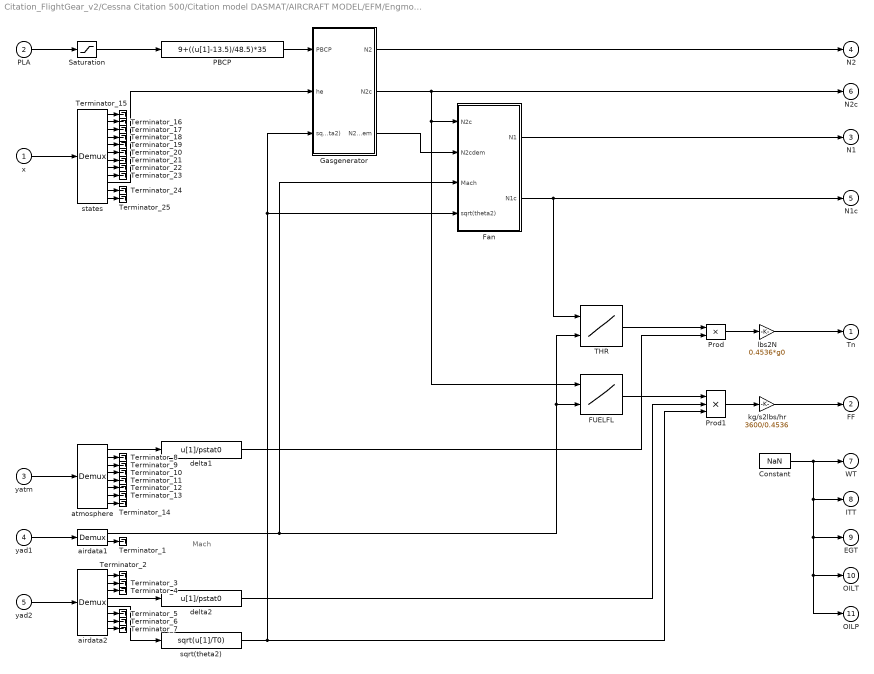
== system Citation_FlightGear_v2/Cessna Citation 500/Citation model DASMAT/AIRCRAFT MODEL/EFM/Engmod/Citation eng_mod/Subsystem1/JT15 Dynamic/Subsystem/engine ==
  note: Mach
  x : Inport
  PLA : Inport  Port=2
  yatm : Inport  Port=3
  yad1 : Inport  Port=4
  yad2 : Inport  Port=5
  Constant : Constant  Value=NaN
  FUELFL : Lookup2D  RowIndex=matff(2:14,1)  ColumnIndex=matff(1,2:14)  Table=matff(2:14,2:14)
  Fan : Subsystem
  Gasgenerator : Subsystem
  PBCP : Fcn  Expr=9+((u[1]-13.5)/48.5)*35
  Prod : Product  InputSameDT=on  SaturateOnIntegerOverflow=on  OutDataTypeStr=Inherit: Same as first input
  Prod1 : Product  Inputs=3  InputSameDT=on  SaturateOnIntegerOverflow=on  OutDataTypeStr=Inherit: Same as first input
  Saturation : Saturate  UpperLimit=62  LowerLimit=13.5
  THR : Lookup2D  RowIndex=matthr(2:12,1)  ColumnIndex=matthr(1,2:12)  Table=matthr(2:12,2:12)
  Terminator_{1..25} (25 alike) : Terminator
  airdata1 : Demux  Outputs=2
      settings: DisplayOption=none
  airdata2 : Demux  Outputs=8
      settings: DisplayOption=none
  atmosphere : Demux  Outputs=8
      settings: DisplayOption=none
  delta1 : Fcn  Expr=u[1]/pstat0
  delta2 : Fcn  Expr=u[1]/pstat0
  kg/s2lbs/hr : Gain  Gain=3600/0.4536  SaturateOnIntegerOverflow=on  OutDataTypeStr=Inherit: Same as input  ParamDataTypeStr=Inherit: Same as input
  lbs2N : Gain  Gain=0.4536*g0  SaturateOnIntegerOverflow=on  OutDataTypeStr=Inherit: Same as input  ParamDataTypeStr=Inherit: Same as input
  sqrt(theta2) : Fcn  Expr=sqrt(u[1]/T0)
  states : Demux  Outputs=12
      settings: DisplayOption=none
  Tn : Outport
  FF : Outport  Port=2
  N1 : Outport  Port=3
  N2 : Outport  Port=4
  N1c : Outport  Port=5
  N2c : Outport  Port=6
  WT : Outport  Port=7
  ITT : Outport  Port=8
  EGT : Outport  Port=9
  OILT : Outport  Port=10
  OILP : Outport  Port=11
  wires:
  states/12 -> Terminator_25/1
  states/11 -> Terminator_24/1
  states/9 -> Terminator_23/1
  states/8 -> Terminator_22/1
  states/7 -> Terminator_21/1
  states/6 -> Terminator_20/1
  states/5 -> Terminator_19/1
  states/4 -> Terminator_18/1
  states/3 -> Terminator_17/1
  states/2 -> Terminator_16/1
  states/1 -> Terminator_15/1
  atmosphere/8 -> Terminator_14/1
  atmosphere/7 -> Terminator_13/1
  atmosphere/6 -> Terminator_12/1
  atmosphere/5 -> Terminator_11/1
  atmosphere/4 -> Terminator_10/1
  atmosphere/3 -> Terminator_9/1
  atmosphere/2 -> Terminator_8/1
  airdata2/8 -> Terminator_7/1
  airdata2/7 -> Terminator_6/1
  airdata2/6 -> Terminator_5/1
  airdata2/3 -> Terminator_4/1
  airdata2/2 -> Terminator_3/1
  airdata2/1 -> Terminator_2/1
  airdata1/2 -> Terminator_1/1
  Fan/2(N1c) -> THR/1, N1c/1
  Gasgenerator/2(N2c) -> Fan/1(N2c), FUELFL/1, N2c/1
  Gasgenerator/3(N2cdem) -> Fan/2(N2cdem)
  airdata1/1 -> Fan/3(Mach), FUELFL/2, THR/2
  Fan/1(N1) -> N1/1
  sqrt(theta2)/1 -> Fan/4(sqrt(theta2)), Gasgenerator/3(sqrt(theta2)), Prod1/3
  yad2/1 -> airdata2/1
  yad1/1 -> airdata1/1
  yatm/1 -> atmosphere/1
  airdata2/4 -> delta2/1
  airdata2/5 -> sqrt(theta2)/1
  Constant/1 -> ITT/1, EGT/1, OILT/1, OILP/1, WT/1
  Gasgenerator/1(N2) -> N2/1
  delta1/1 -> Prod/2
  Prod/1 -> lbs2N/1
  THR/1 -> Prod/1
  lbs2N/1 -> Tn/1
  states/10 -> Gasgenerator/2(he)
  delta2/1 -> Prod1/2
  atmosphere/1 -> delta1/1
  Prod1/1 -> kg/s2lbs/hr/1
  kg/s2lbs/hr/1 -> FF/1
  Saturation/1 -> PBCP/1
  PLA/1 -> Saturation/1
  x/1 -> states/1
  PBCP/1 -> Gasgenerator/1(PBCP)
  FUELFL/1 -> Prod1/1

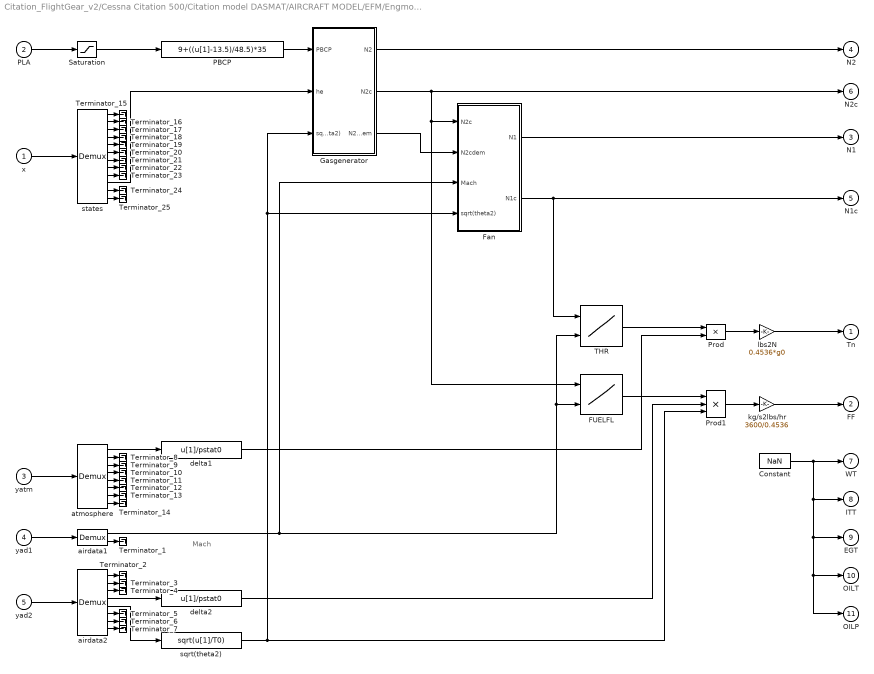
== system Citation_FlightGear_v2/Cessna Citation 500/Citation model DASMAT/AIRCRAFT MODEL/EFM/Engmod/Citation eng_mod/Subsystem1/JT15 Dynamic1/Subsystem/engine ==
  note: Mach
  x : Inport
  PLA : Inport  Port=2
  yatm : Inport  Port=3
  yad1 : Inport  Port=4
  yad2 : Inport  Port=5
  Constant : Constant  Value=NaN
  FUELFL : Lookup2D  RowIndex=matff(2:14,1)  ColumnIndex=matff(1,2:14)  Table=matff(2:14,2:14)
  Fan : Subsystem
  Gasgenerator : Subsystem
  PBCP : Fcn  Expr=9+((u[1]-13.5)/48.5)*35
  Prod : Product  InputSameDT=on  SaturateOnIntegerOverflow=on  OutDataTypeStr=Inherit: Same as first input
  Prod1 : Product  Inputs=3  InputSameDT=on  SaturateOnIntegerOverflow=on  OutDataTypeStr=Inherit: Same as first input
  Saturation : Saturate  UpperLimit=62  LowerLimit=13.5
  THR : Lookup2D  RowIndex=matthr(2:12,1)  ColumnIndex=matthr(1,2:12)  Table=matthr(2:12,2:12)
  Terminator_{1..25} (25 alike) : Terminator
  airdata1 : Demux  Outputs=2
      settings: DisplayOption=none
  airdata2 : Demux  Outputs=8
      settings: DisplayOption=none
  atmosphere : Demux  Outputs=8
      settings: DisplayOption=none
  delta1 : Fcn  Expr=u[1]/pstat0
  delta2 : Fcn  Expr=u[1]/pstat0
  kg/s2lbs/hr : Gain  Gain=3600/0.4536  SaturateOnIntegerOverflow=on  OutDataTypeStr=Inherit: Same as input  ParamDataTypeStr=Inherit: Same as input
  lbs2N : Gain  Gain=0.4536*g0  SaturateOnIntegerOverflow=on  OutDataTypeStr=Inherit: Same as input  ParamDataTypeStr=Inherit: Same as input
  sqrt(theta2) : Fcn  Expr=sqrt(u[1]/T0)
  states : Demux  Outputs=12
      settings: DisplayOption=none
  Tn : Outport
  FF : Outport  Port=2
  N1 : Outport  Port=3
  N2 : Outport  Port=4
  N1c : Outport  Port=5
  N2c : Outport  Port=6
  WT : Outport  Port=7
  ITT : Outport  Port=8
  EGT : Outport  Port=9
  OILT : Outport  Port=10
  OILP : Outport  Port=11
  wires:
  states/12 -> Terminator_25/1
  states/11 -> Terminator_24/1
  states/9 -> Terminator_23/1
  states/8 -> Terminator_22/1
  states/7 -> Terminator_21/1
  states/6 -> Terminator_20/1
  states/5 -> Terminator_19/1
  states/4 -> Terminator_18/1
  states/3 -> Terminator_17/1
  states/2 -> Terminator_16/1
  states/1 -> Terminator_15/1
  atmosphere/8 -> Terminator_14/1
  atmosphere/7 -> Terminator_13/1
  atmosphere/6 -> Terminator_12/1
  atmosphere/5 -> Terminator_11/1
  atmosphere/4 -> Terminator_10/1
  atmosphere/3 -> Terminator_9/1
  atmosphere/2 -> Terminator_8/1
  airdata2/8 -> Terminator_7/1
  airdata2/7 -> Terminator_6/1
  airdata2/6 -> Terminator_5/1
  airdata2/3 -> Terminator_4/1
  airdata2/2 -> Terminator_3/1
  airdata2/1 -> Terminator_2/1
  airdata1/2 -> Terminator_1/1
  Fan/2(N1c) -> THR/1, N1c/1
  Gasgenerator/2(N2c) -> Fan/1(N2c), FUELFL/1, N2c/1
  Gasgenerator/3(N2cdem) -> Fan/2(N2cdem)
  airdata1/1 -> Fan/3(Mach), FUELFL/2, THR/2
  Fan/1(N1) -> N1/1
  sqrt(theta2)/1 -> Fan/4(sqrt(theta2)), Gasgenerator/3(sqrt(theta2)), Prod1/3
  yad2/1 -> airdata2/1
  yad1/1 -> airdata1/1
  yatm/1 -> atmosphere/1
  airdata2/4 -> delta2/1
  airdata2/5 -> sqrt(theta2)/1
  Constant/1 -> ITT/1, EGT/1, OILT/1, OILP/1, WT/1
  Gasgenerator/1(N2) -> N2/1
  delta1/1 -> Prod/2
  Prod/1 -> lbs2N/1
  THR/1 -> Prod/1
  lbs2N/1 -> Tn/1
  states/10 -> Gasgenerator/2(he)
  delta2/1 -> Prod1/2
  atmosphere/1 -> delta1/1
  Prod1/1 -> kg/s2lbs/hr/1
  kg/s2lbs/hr/1 -> FF/1
  Saturation/1 -> PBCP/1
  PLA/1 -> Saturation/1
  x/1 -> states/1
  PBCP/1 -> Gasgenerator/1(PBCP)
  FUELFL/1 -> Prod1/1

== system Citation_FlightGear_v2/Cessna Citation 500/Citation model DASMAT/AIRCRAFT MODEL/EFM/Engmod/Citation eng_mod/Subsystem1/JT15 Dynamic/Subsystem/engine/Fan ==
  note: N1c feedback
  note: N1cdot
  N2c : Inport
  N2cdem : Inport  Port=2
  Mach : Inport  Port=3
  sqrt(theta2) : Inport  Port=4
  Droop : Gain  Gain=2  SaturateOnIntegerOverflow=on  OutDataTypeStr=Inherit: Same as input  ParamDataTypeStr=Inherit: Same as input
  Max accel : Subsystem  mask(Min Value){}
      mask help:
      | Output is minimum value of inputs.
      | y=min(u1,u2)
      mask Help: The Min block produces as output the minimum value of two scalars or vectors. If the inputs are vectors, the output will be a vector containing the minimum elements of the vectors.
      mask Display: disp('Min')
  Max decel : Subsystem  mask(Max Value){}
      mask help:
      | Output is maximum value of inputs.
      | y=max(u1,u2)
      mask Help: The Max block produces as output the maximum value of two scalars or vectors. If the inputs are vectors, the output will be a vector containing the maximum elements of the vectors.
      mask Display: disp('Max')
  N1 state : Integrator  InitialCondition=xt0(2)
  N1D : Lookup2D  RowIndex=matn1d(2:14,1)  ColumnIndex=matn1d(1,2:14)  Table=matn1d(2:14,2:14)
  Prod : Product  InputSameDT=on  SaturateOnIntegerOverflow=on  OutDataTypeStr=Inherit: Same as first input
  Sum : Sum  Inputs=+-  InputSameDT=on  SaturateOnIntegerOverflow=on  OutDataTypeStr=Inherit: Same as first input
  fN1cmax : Lookup  InputValues="[0 25 40 70 94  120]"  Table="[0   0   1   12 14  18]"
  fN1cmin : Lookup  InputValues="[25     50   60   94 100]"  Table="[-0.05  -0.05    -1    -30 -28]"
  N1 : Outport
  N1c : Outport  Port=2
  wires:
  sqrt(theta2)/1 -> Prod/2
  N1 state/1 -> Prod/1, Sum/2, N1c/1
  N2c/1 -> fN1cmin/1, fN1cmax/1
  Max decel/1(out_1) -> N1 state/1
  N1D/1 -> Sum/1
  Max accel/1(out_1) -> Max decel/1(in_1)
  fN1cmax/1 -> Max accel/2(in_2)
  fN1cmin/1 -> Max decel/2(in_2)
  Sum/1 -> Droop/1
  Droop/1 -> Max accel/1(in_1)
  Mach/1 -> N1D/2
  Prod/1 -> N1/1
  N2cdem/1 -> N1D/1

== system Citation_FlightGear_v2/Cessna Citation 500/Citation model DASMAT/AIRCRAFT MODEL/EFM/Engmod/Citation eng_mod/Subsystem1/JT15 Dynamic/Subsystem/engine/Gasgenerator ==
  note: N2 feedback
  note: N2dot
  PBCP : Inport
  he : Inport  Port=2
  sqrt(theta2) : Inport  Port=3
  Droop : Lookup  InputValues=[0 100]  Table="[0.1  2]"
  Fcn : Fcn  Expr=u[1]/u[2]
  Fcn1 : Fcn  Expr=u[1]/u[2]
  Governor : Product  InputSameDT=on  SaturateOnIntegerOverflow=on  OutDataTypeStr=Inherit: Same as first input
  Max accel : Subsystem  mask(Max Value){}
      mask help:
      | Output is maximum value of inputs.
      | y=max(u1,u2)
      mask Help: The Max block produces as output the maximum value of two scalars or vectors. If the inputs are vectors, the output will be a vector containing the maximum elements of the vectors.
      mask Display: disp('Max')
  Min accel : Subsystem  mask(Min Value){}
      mask help:
      | Output is minimum value of inputs.
      | y=min(u1,u2)
      mask Help: The Min block produces as output the minimum value of two scalars or vectors. If the inputs are vectors, the output will be a vector containing the minimum elements of the vectors.
      mask Display: disp('Min')
  Mux : Mux  Inputs=2
  Mux1 : Mux  Inputs=2
  N2 state : Integrator  InitialCondition=xt0(1)
  N2D : Lookup2D  RowIndex=matn2d(2:10,1)  ColumnIndex=matn2d(1,2:10)  Table=matn2d(2:10,2:10)
  Sum : Sum  Inputs=+-  InputSameDT=on  SaturateOnIntegerOverflow=on  OutDataTypeStr=Inherit: Same as first input
  fN2max : Lookup  InputValues=[25 40 70 94]  Table=[0 3 8 10]
  fN2min : Lookup  InputValues="[25     50   60   94 100]"  Table="[-0.05  -0.05    -2    -20 -28]"
  ft2FL : Gain  Gain=.01  SaturateOnIntegerOverflow=on  OutDataTypeStr=Inherit: Same as input  ParamDataTypeStr=Inherit: Same as input
  m2ft : Gain  Gain=(1/0.3048)  SaturateOnIntegerOverflow=on  OutDataTypeStr=Inherit: Same as input  ParamDataTypeStr=Inherit: Same as input
  N2 : Outport
  N2c : Outport  Port=2
  N2cdem : Outport  Port=3
  wires:
  sqrt(theta2)/1 -> Mux1/2, Mux/2
  N2D/1 -> Mux/1, Droop/1, Sum/1
  Fcn1/1 -> N2c/1
  Fcn/1 -> N2cdem/1
  Mux1/1 -> Fcn1/1
  Mux/1 -> Fcn/1
  Min accel/1(out_1) -> Max accel/1(in_1)
  ft2FL/1 -> N2D/2
  m2ft/1 -> ft2FL/1
  he/1 -> m2ft/1
  N2 state/1 -> Mux1/1, fN2min/1, fN2max/1, Sum/2, N2/1
  fN2max/1 -> Min accel/2(in_2)
  fN2min/1 -> Max accel/2(in_2)
  PBCP/1 -> N2D/1
  Droop/1 -> Governor/1
  Sum/1 -> Governor/2
  Governor/1 -> Min accel/1(in_1)
  Max accel/1(out_1) -> N2 state/1

== system Citation_FlightGear_v2/Cessna Citation 500/Citation model DASMAT/AIRCRAFT MODEL/EFM/Engmod/Citation eng_mod/Subsystem1/JT15 Dynamic1/Subsystem/engine/Fan ==
  note: N1c feedback
  note: N1cdot
  N2c : Inport
  N2cdem : Inport  Port=2
  Mach : Inport  Port=3
  sqrt(theta2) : Inport  Port=4
  Droop : Gain  Gain=2  SaturateOnIntegerOverflow=on  OutDataTypeStr=Inherit: Same as input  ParamDataTypeStr=Inherit: Same as input
  Max accel : Subsystem  mask(Min Value){}
      mask help:
      | Output is minimum value of inputs.
      | y=min(u1,u2)
      mask Help: The Min block produces as output the minimum value of two scalars or vectors. If the inputs are vectors, the output will be a vector containing the minimum elements of the vectors.
      mask Display: disp('Min')
  Max decel : Subsystem  mask(Max Value){}
      mask help:
      | Output is maximum value of inputs.
      | y=max(u1,u2)
      mask Help: The Max block produces as output the maximum value of two scalars or vectors. If the inputs are vectors, the output will be a vector containing the maximum elements of the vectors.
      mask Display: disp('Max')
  N1 state : Integrator  InitialCondition=xt0(2)
  N1D : Lookup2D  RowIndex=matn1d(2:14,1)  ColumnIndex=matn1d(1,2:14)  Table=matn1d(2:14,2:14)
  Prod : Product  InputSameDT=on  SaturateOnIntegerOverflow=on  OutDataTypeStr=Inherit: Same as first input
  Sum : Sum  Inputs=+-  InputSameDT=on  SaturateOnIntegerOverflow=on  OutDataTypeStr=Inherit: Same as first input
  fN1cmax : Lookup  InputValues="[0 25 40 70 94  120]"  Table="[0   0   1   12 14  18]"
  fN1cmin : Lookup  InputValues="[25     50   60   94 100]"  Table="[-0.05  -0.05    -1    -30 -28]"
  N1 : Outport
  N1c : Outport  Port=2
  wires:
  sqrt(theta2)/1 -> Prod/2
  N1 state/1 -> Prod/1, Sum/2, N1c/1
  N2c/1 -> fN1cmin/1, fN1cmax/1
  Max decel/1(out_1) -> N1 state/1
  N1D/1 -> Sum/1
  Max accel/1(out_1) -> Max decel/1(in_1)
  fN1cmax/1 -> Max accel/2(in_2)
  fN1cmin/1 -> Max decel/2(in_2)
  Sum/1 -> Droop/1
  Droop/1 -> Max accel/1(in_1)
  Mach/1 -> N1D/2
  Prod/1 -> N1/1
  N2cdem/1 -> N1D/1
